simulink model "tuningvaluesmodel"  (Simulink 10.0)
settings: Solver=ode45  StartTime=0.0  StopTime=1500  RelTol=1e-3  EnableMultiTasking=on
undefined symbols (not defined in the file): ctrl, intgrl, var
libraries: simulink x2
settings Model: Creator=MAHE  LastModifiedBy=fasee
settings DataIOCC: LimitDataPoints=on
settings DebuggingCC: UnderspecifiedInitializationDetection=Simplified  MergeDetectMultiDrivingBlocksExec=error  SolverPrmCheckMsg=warning  UnderSpecifiedDimensionMsg=warning
settings GRTTargetCC: GeneratePreprocessorConditionals=Disable all  CombineOutputUpdateFcns=on  GRTInterface=off
settings ConfigComp: CovExternalEMLEnable=off  CovSFcnEnable=off

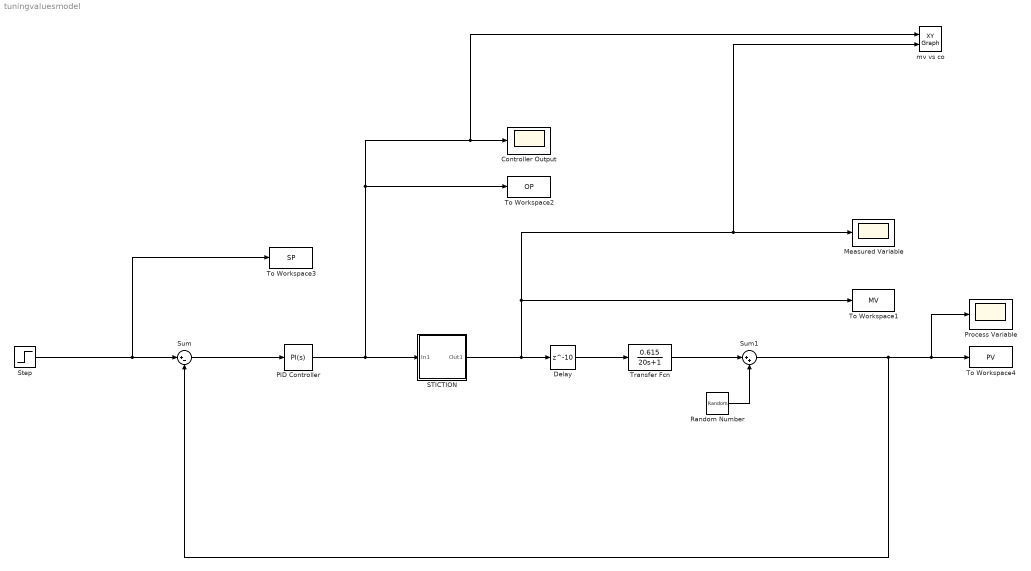
== system tuningvaluesmodel ==
  Controller Output : Scope
  Delay : Delay  DelayLength=10  InitialCondition=0
  Measured Variable : Scope
  PID Controller : simulink/Continuous/PID Controller  Controller=PI  Form=Parallel  TimeDomain=Continuous-time  SampleTime=-1  IntegratorMethod=Forward Euler  FilterMethod=Forward Euler  ControllerParametersSource=internal  P=ctrl  I=intgrl  D=0  UseFilter=on  N=100  TunerSelectOption=Transfer Function Based (PID Tuner App)  InitialConditionSource=internal  InitialConditionForIntegrator=0  InitialConditionForFilter=0  DifferentiatorICPrevScaledInput=0  ExternalReset=none  TrackingMode=off  Kt=1  LimitOutput=off  UpperSaturationLimit=inf  LowerSaturationLimit=-inf  LinearizeAsGain=on  AntiWindupMode=none  Kb=1  POutMin=[]  POutMax=[]  IOutMin=[]  IOutMax=[]  DOutMin=[]  DOutMax=[]  NOutMin=[]  NOutMax=[]  SumOutMin=[]  SumOutMax=[]  SaturationOutMin=[]  SaturationOutMax=[]  PParamMin=[]  PParamMax=[]  IParamMin=[]  IParamMax=[]  DParamMin=[]  DParamMax=[]  NParamMin=[]  NParamMax=[]  KbParamMin=[]  KbParamMax=[]  KtParamMin=[]  KtParamMax=[]  KbOutMin=[]  KbOutMax=[]  KtOutMin=[]  KtOutMax=[]  IntegratorOutMin=[]  IntegratorOutMax=[]  FilterOutMin=[]  FilterOutMax=[]  SumI1OutMin=[]  SumI1OutMax=[]  SumI2OutMin=[]  SumI2OutMax=[]  SumI3OutMin=[]  SumI3OutMax=[]  SumI4OutMin=[]  SumI4OutMax=[]  SumDOutMin=[]  SumDOutMax=[]  DifferentiatorOutMin=[]  DifferentiatorOutMax=[]  FilterDiffOutCoefMin=[]  FilterDiffOutCoefMax=[]  ReciprocalOutMin=[]  ReciprocalOutMax=[]  SumDenOutMin=[]  SumDenOutMax=[]  SumNumOutMin=[]  SumNumOutMax=[]  DivideOutMin=[]  DivideOutMax=[]  IntegratorContinuousStateAttributes=''  IntegratorStateMustResolveToSignalObject=off  IntegratorRTWStateStorageClass=Auto  FilterContinuousStateAttributes=''  FilterStateMustResolveToSignalObject=off  FilterRTWStateStorageClass=Auto  ParallelPVariant=InternalParameters  IdealPVariant=Disabled  IVariant=InternalParameters  DVariant=Disabled  IntegratorVariant=Continuous  SatVariant=Disabled  AWVariant=Passthrough  PCopyVariant=Disabled  TRVariant=Disabled  FdbkBlocksVariant=Forward  IdealPFdbkVariant=Disabled  SatFdbkVariant=Disabled  DerivativeFilterVariant=Disabled  NVariant=Disabled  NCopyVariant=Disabled_SignalSpec  FilterICVariant=Disabled  IntegratorICVariant=InternalICs  ExternalResetVariant=Disabled  TRSumVariant=Passthrough  SumFdbkVariant=Disabled  SumVariant=Sum_PI
  Process Variable : Scope
  Random Number : RandomNumber  Variance=var  SampleTime=1
  STICTION : Subsystem
  Step : Step  Time=50  After=30  SampleTime=1
  Sum : Sum  Inputs=|+-
  Sum1 : Sum  Inputs=|++
  To Workspace1 : ToWorkspace  VariableName=MV  SampleTime=-1
  To Workspace2 : ToWorkspace  VariableName=OP  SampleTime=-1
  To Workspace3 : ToWorkspace  VariableName=SP  SampleTime=-1
  To Workspace4 : ToWorkspace  VariableName=PV  SampleTime=-1
  Transfer Fcn : TransferFcn  Numerator=[0.615]  Denominator=[20 1]
  mv vs co : simulink/Sinks/XY Graph  xmin=-100  xmax=100  ymin=-100  ymax=100  st=1
  wires:
  Step/1 -> To Workspace3/1, Sum/1
  Sum/1 -> PID Controller/1
  PID Controller/1 -> STICTION/1(In1), mv vs co/1, Controller Output/1, To Workspace2/1
  Random Number/1 -> Sum1/2
  STICTION/1(Out1) -> Delay/1, mv vs co/2, Measured Variable/1, To Workspace1/1
  Delay/1 -> Transfer Fcn/1
  Transfer Fcn/1 -> Sum1/1
  Sum1/1 -> Sum/2, Process Variable/1, To Workspace4/1

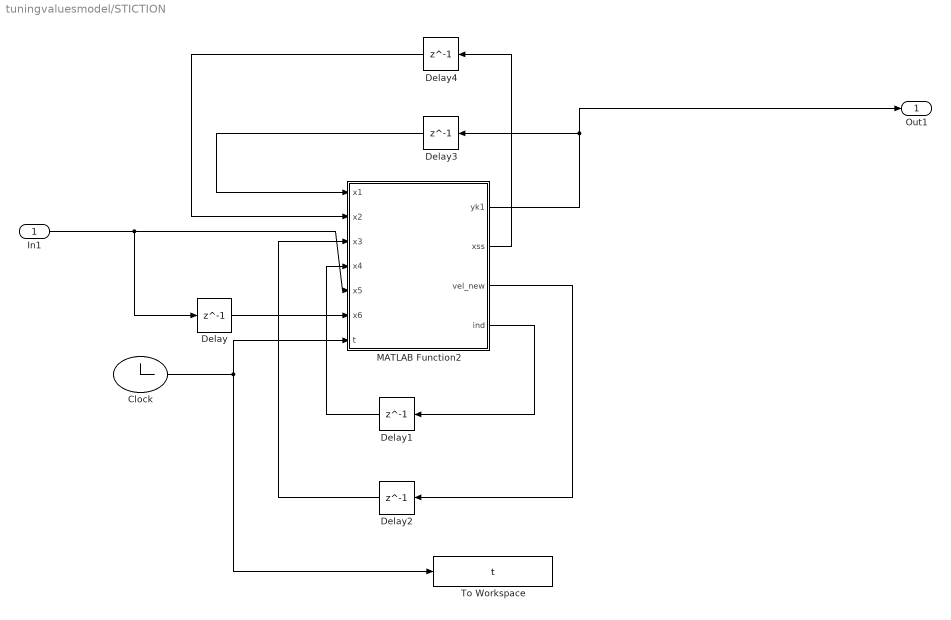
== system tuningvaluesmodel/STICTION ==
  In1 : Inport
  Clock : Clock
  Delay{,1,3..4} (4 alike) : Delay  DelayLength=1  InitialCondition=0  SampleTime=1
  Delay2 : Delay  DelayLength=1  InitialCondition=0
  MATLAB Function2 : MATLAB Function  TreatAsAtomicUnit=on
  To Workspace : ToWorkspace  VariableName=t  SampleTime=1
  Out1 : Outport
  wires:
  Delay4/1 -> MATLAB Function2/2(x2)
  Delay/1 -> MATLAB Function2/6(x6)
  MATLAB Function2/1(yk1) -> Out1/1, Delay3/1
  Delay1/1 -> MATLAB Function2/4(x4)
  Clock/1 -> To Workspace/1, MATLAB Function2/7(t)
  In1/1 -> Delay/1, MATLAB Function2/5(x5)
  MATLAB Function2/3(vel_new) -> Delay2/1
  Delay2/1 -> MATLAB Function2/3(x3)
  MATLAB Function2/4(ind) -> Delay1/1
  Delay3/1 -> MATLAB Function2/1(x1)
  MATLAB Function2/2(xss) -> Delay4/1

== matlab function STICTION/MATLAB Function2 ==
  data: x1 input double; yk1 output double; x2 input double; x3 input double; x4 input double; x5 input double; x6 input double; xss output double; vel_new output double; t input double; ind output double
function [yk1,xss,vel_new,ind] = StictionModel(x1,x2,x3,x4,x5,x6,t)
S = 0;
j = 0;
delta_t=1; 

    
if t==0
   vel_old=0.01;
   xss=0;
   yk=0;
   xk=0;
   xk1=x5;
   ind=0;
   
else
    yk=x1;
    xss=x2; 
    xk=x6;
    xk1=x5; %(100*sin(2*pi*0.01*(t))+100)/2
    vel_old=x3;
    ind = x4;
end
    
vel_new=(xk1-xk)/delta_t; 

    if S==0&&j==0
        yk1=xk1;


    else
        if xk1>100
            yk1=100;
            xss=100;
        else
            if xk1<0
                yk1=0;
                xss=0;
            else
                if (sign(vel_old)~=sign(vel_new));
                    if sign(vel_new)~=0 
                        xss=xk;
                        yk1=yk; 
                    else
                        ind=1;
                        xss=xk;
                        yk1=yk;                                  
                    end
                else
                    if ind~=1
                            if abs(xk1-xss)>S
                                %yk1=xk1-sign(vel_new)*S/2+sign(vel_new)*jump/2;
                                yk1 = xk1 - ((sign(vel_new))*((S-j)/2));
                            else
                                yk1=yk; 
                            end 
                    else
                        if abs(xk1-xss)>j 
                            %yk1=xk1-sign(vel_new)*S/2+sign(vel_new)*jump/2;  
                            ind=0;
                            yk1 = xk1 - ((sign(vel_new))*((S-j)/2));
                        else
                            yk1=yk;
                        end
                    end
                end
            end
        end

    end
    

end
